simulink model "regulator_LQR_discrete"  (R2021b)
settings: Solver=VariableStepAuto  StartTime=0.0  StopTime=10.0  RelTol=1e-3
values from neighbouring files (symbols this model uses):
  C_temp = eye(length(A))    [main3.m]
  D_temp = zeros(length(B), 1)    [main3.m]
  LQ_d = dlqr(A,B,Q,R)    [main3.m]
  LQ_d2 = dlqr(A,B,Q_2,R_2)    [main3.m]
  U_bar = Y_bar / G_1    [main3.m]
  x_0 = [5 20]'    [main3.m]
  X_bar = inv(eye(2)-A)*B*U_bar    [main3.m]
undefined symbols (not defined in the file or in its folder): A, B, C
settings Model: Creator=PaoloA  LastModifiedBy=PaoloA

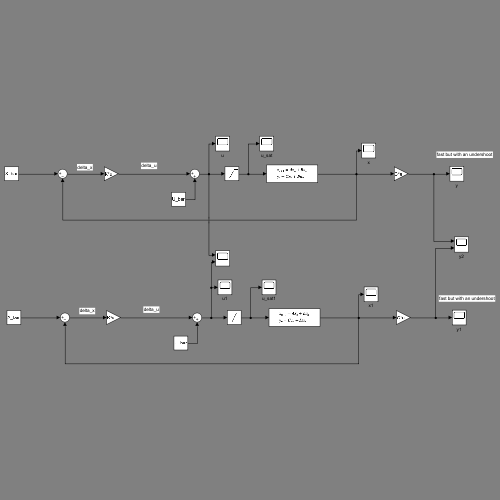
[thumbnail: Simulink's stored preview of the top-level diagram]
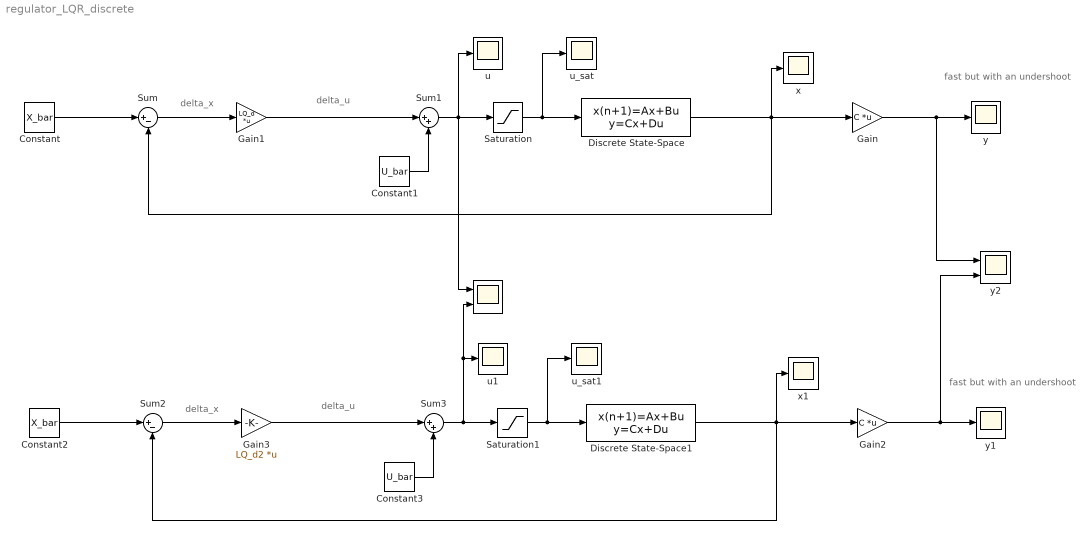
== system regulator_LQR_discrete ==
  note: fast but with an undershoot
  note: delta_u
  note: delta_x
  note: delta_u
  note: delta_x
  note: fast but with an undershoot
  " " : Scope  NumInputPorts=2
  Constant : Constant  Value=X_bar
  Constant1 : Constant  Value=U_bar
  Constant2 : Constant  Value=X_bar
  Constant3 : Constant  Value=U_bar
  Discrete State-Space : DiscreteStateSpace  A=A  B=B  C=C_temp  D=D_temp  InitialCondition=x_0  SampleTime=-1
  Discrete State-Space1 : DiscreteStateSpace  A=A  B=B  C=C_temp  D=D_temp  InitialCondition=x_0  SampleTime=-1
  Gain : Gain  Gain=C  Multiplication=Matrix(K*u)
  Gain1 : Gain  Gain=LQ_d  Multiplication=Matrix(K*u)
  Gain2 : Gain  Gain=C  Multiplication=Matrix(K*u)
  Gain3 : Gain  Gain=LQ_d2  Multiplication=Matrix(K*u)
  Saturation : Saturate  UpperLimit=+inf  LowerLimit=-inf
  Saturation1 : Saturate  UpperLimit=+inf  LowerLimit=-inf
  Sum : Sum  Inputs=|+-
  Sum1 : Sum  Inputs=|++
  Sum2 : Sum  Inputs=|+-
  Sum3 : Sum  Inputs=|++
  u : Scope
  u1 : Scope
  u_sat : Scope
  u_sat1 : Scope
  x : Scope
  x1 : Scope
  y : Scope
  y1 : Scope
  y2 : Scope  NumInputPorts=2
  wires:
  Constant/1 -> Sum/1
  Sum/1 -> Gain1/1
  Gain1/1 -> Sum1/1
  Constant1/1 -> Sum1/2
  Sum1/1 -> " "/1, u/1, Saturation/1
  Saturation/1 -> u_sat/1, Discrete State-Space/1
  Discrete State-Space/1 -> x/1, Gain/1, Sum/2
  Gain/1 -> y2/1, y/1
  Saturation1/1 -> u_sat1/1, Discrete State-Space1/1
  Gain2/1 -> y2/2, y1/1
  Sum3/1 -> " "/2, u1/1, Saturation1/1
  Discrete State-Space1/1 -> x1/1, Gain2/1, Sum2/2
  Constant2/1 -> Sum2/1
  Gain3/1 -> Sum3/1
  Sum2/1 -> Gain3/1
  Constant3/1 -> Sum3/2
